simulink model "TCT_and_SUDOKU"  (R2025a)
settings: Solver=VariableStepAuto  StartTime=0.0  StopTime=1  RelTol=1e-3
libraries: spsDiodeLib x162, spsPVArrayLib x162, spsControlledVoltageSourceLib x2, spsCurrentMeasurementLib x2, simulink x2, spsVoltageMeasurementLib x2, sps_lib x1
(part 2 of 2)

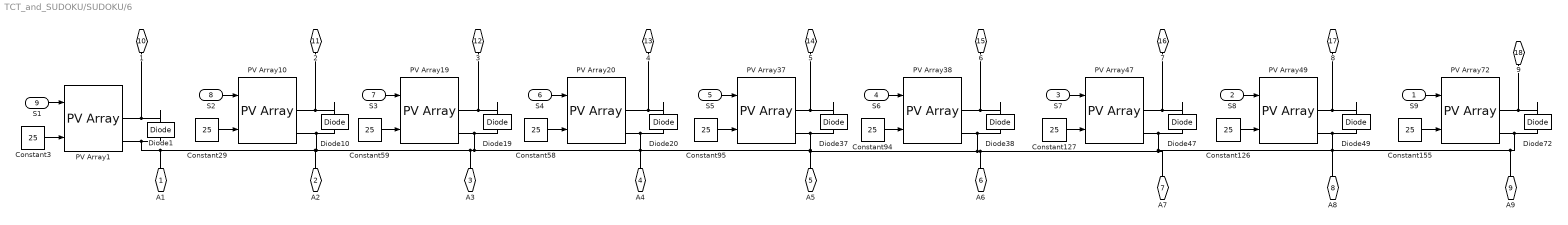
== system TCT_and_SUDOKU/SUDOKU/6 ==
  S9 : Inport
  S8 : Inport  Port=2
  S7 : Inport  Port=3
  S6 : Inport  Port=4
  S5 : Inport  Port=5
  S4 : Inport  Port=6
  S3 : Inport  Port=7
  S2 : Inport  Port=8
  S1 : Inport  Port=9
  Constant{3,29,58..59,94..95,126..127,155} (9 alike) : Constant  Value=25
  Diode{1,10,19..20,37..38,47,49,72} (9 alike) : spsDiodeLib/Diode  Ron=0.001  Lon=0  Vf=0.8  IC=0  UseSnubber=0  Rs=500  Cs=250e-9  Measurements=off
  PV Array{1,10,19..20,37..38,47,49,72} (9 alike) : spsPVArrayLib/PV Array  Npar=1  Nser=1  PlotType=array @ 1000 W/m2 & specified temperatures  S_vec="[ 1000  500  100 ]"  Temp_C_vec="[ 45 25  ]"  ModuleName=User-defined  PlotWhenSelected=off  Pm=79.2  Ncell=60  Voc=22  Isc=4.7  Vm=18  Im=4.4  beta_Voc_pc=-0.36099  alpha_Isc_pc=0.102  beta_Voc=-0.079418  alpha_Isc=0.004794  IL=4.7103  I0=1.7336e-10  nI=0.59447  Rsh=255.4401  Rs=0.29081  RobustModel=off  RobustCellTemperature=313.3991  BAL=on  Tc=1e-6  Tfilter=5e-5
  A1 : PMIOPort  Side=Left
  A2 : PMIOPort  Port=2  Side=Left
  A3 : PMIOPort  Port=3  Side=Left
  A4 : PMIOPort  Port=4  Side=Left
  A5 : PMIOPort  Port=5  Side=Left
  A6 : PMIOPort  Port=6  Side=Left
  A7 : PMIOPort  Port=7  Side=Left
  A8 : PMIOPort  Port=8  Side=Left
  A9 : PMIOPort  Port=9  Side=Left
  1 : PMIOPort  Port=10  Side=Right
  2 : PMIOPort  Port=11  Side=Right
  3 : PMIOPort  Port=12  Side=Right
  4 : PMIOPort  Port=13  Side=Right
  5 : PMIOPort  Port=14  Side=Right
  6 : PMIOPort  Port=15  Side=Right
  7 : PMIOPort  Port=16  Side=Right
  8 : PMIOPort  Port=17  Side=Right
  9 : PMIOPort  Port=18  Side=Right
  wires:
  S2/1 -> PV Array10/1
  S3/1 -> PV Array19/1
  Constant3/1 -> PV Array1/2
  S9/1 -> PV Array72/1
  Constant59/1 -> PV Array19/2
  Constant58/1 -> PV Array20/2
  Constant29/1 -> PV Array10/2
  Constant155/1 -> PV Array72/2
  S4/1 -> PV Array20/1
  S8/1 -> PV Array49/1
  Constant94/1 -> PV Array38/2
  Constant127/1 -> PV Array47/2
  S5/1 -> PV Array37/1
  Constant95/1 -> PV Array37/2
  S1/1 -> PV Array1/1
  S6/1 -> PV Array38/1
  Constant126/1 -> PV Array49/2
  S7/1 -> PV Array47/1
  connections:
  Diode10/RConn1 -- 2/RConn1 -- PV Array10/RConn1
  Diode20/RConn1 -- 4/RConn1 -- PV Array20/RConn1
  Diode19/RConn1 -- 3/RConn1 -- PV Array19/RConn1
  A6/RConn1 -- Diode47/LConn1 -- PV Array47/RConn2 -- A8/RConn1 -- Diode72/LConn1 -- PV Array72/RConn2 -- A9/RConn1 -- Diode49/LConn1 -- PV Array49/RConn2 -- A7/RConn1 -- Diode37/LConn1 -- PV Array37/RConn2 -- PV Array1/RConn2 -- Diode1/LConn1 -- A1/RConn1 -- A2/RConn1 -- PV Array10/RConn2 -- Diode10/LConn1 -- A3/RConn1 -- Diode19/LConn1 -- PV Array19/RConn2 -- A4/RConn1 -- Diode20/LConn1 -- PV Array20/RConn2 -- A5/RConn1 -- Diode38/LConn1 -- PV Array38/RConn2
  Diode47/RConn1 -- 7/RConn1 -- PV Array47/RConn1
  Diode49/RConn1 -- PV Array49/RConn1 -- 8/RConn1
  Diode1/RConn1 -- 1/RConn1 -- PV Array1/RConn1
  Diode72/RConn1 -- 9/RConn1 -- PV Array72/RConn1
  Diode37/RConn1 -- PV Array37/RConn1 -- 5/RConn1
  Diode38/RConn1 -- 6/RConn1 -- PV Array38/RConn1

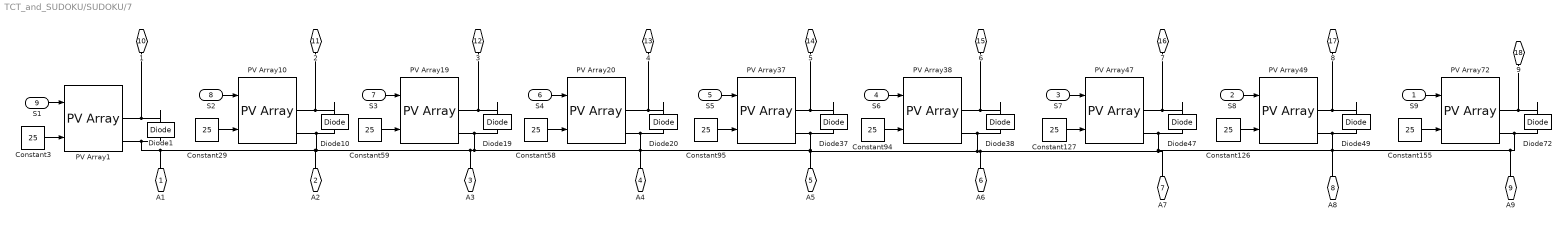
== system TCT_and_SUDOKU/SUDOKU/7 ==
  S9 : Inport
  S8 : Inport  Port=2
  S7 : Inport  Port=3
  S6 : Inport  Port=4
  S5 : Inport  Port=5
  S4 : Inport  Port=6
  S3 : Inport  Port=7
  S2 : Inport  Port=8
  S1 : Inport  Port=9
  Constant{3,29,58..59,94..95,126..127,155} (9 alike) : Constant  Value=25
  Diode{1,10,19..20,37..38,47,49,72} (9 alike) : spsDiodeLib/Diode  Ron=0.001  Lon=0  Vf=0.8  IC=0  UseSnubber=0  Rs=500  Cs=250e-9  Measurements=off
  PV Array{1,10,19..20,37..38,47,49,72} (9 alike) : spsPVArrayLib/PV Array  Npar=1  Nser=1  PlotType=array @ 1000 W/m2 & specified temperatures  S_vec="[ 1000  500  100 ]"  Temp_C_vec="[ 45 25  ]"  ModuleName=User-defined  PlotWhenSelected=off  Pm=79.2  Ncell=60  Voc=22  Isc=4.7  Vm=18  Im=4.4  beta_Voc_pc=-0.36099  alpha_Isc_pc=0.102  beta_Voc=-0.079418  alpha_Isc=0.004794  IL=4.7103  I0=1.7336e-10  nI=0.59447  Rsh=255.4401  Rs=0.29081  RobustModel=off  RobustCellTemperature=313.3991  BAL=on  Tc=1e-6  Tfilter=5e-5
  A1 : PMIOPort  Side=Left
  A2 : PMIOPort  Port=2  Side=Left
  A3 : PMIOPort  Port=3  Side=Left
  A4 : PMIOPort  Port=4  Side=Left
  A5 : PMIOPort  Port=5  Side=Left
  A6 : PMIOPort  Port=6  Side=Left
  A7 : PMIOPort  Port=7  Side=Left
  A8 : PMIOPort  Port=8  Side=Left
  A9 : PMIOPort  Port=9  Side=Left
  1 : PMIOPort  Port=10  Side=Right
  2 : PMIOPort  Port=11  Side=Right
  3 : PMIOPort  Port=12  Side=Right
  4 : PMIOPort  Port=13  Side=Right
  5 : PMIOPort  Port=14  Side=Right
  6 : PMIOPort  Port=15  Side=Right
  7 : PMIOPort  Port=16  Side=Right
  8 : PMIOPort  Port=17  Side=Right
  9 : PMIOPort  Port=18  Side=Right
  wires:
  S7/1 -> PV Array47/1
  Constant126/1 -> PV Array49/2
  S6/1 -> PV Array38/1
  S1/1 -> PV Array1/1
  Constant95/1 -> PV Array37/2
  S5/1 -> PV Array37/1
  Constant127/1 -> PV Array47/2
  Constant94/1 -> PV Array38/2
  S8/1 -> PV Array49/1
  S4/1 -> PV Array20/1
  Constant155/1 -> PV Array72/2
  Constant29/1 -> PV Array10/2
  Constant58/1 -> PV Array20/2
  Constant59/1 -> PV Array19/2
  S9/1 -> PV Array72/1
  Constant3/1 -> PV Array1/2
  S3/1 -> PV Array19/1
  S2/1 -> PV Array10/1
  connections:
  PV Array38/RConn1 -- 6/RConn1 -- Diode38/RConn1
  5/RConn1 -- PV Array37/RConn1 -- Diode37/RConn1
  PV Array72/RConn1 -- 9/RConn1 -- Diode72/RConn1
  PV Array1/RConn1 -- 1/RConn1 -- Diode1/RConn1
  8/RConn1 -- PV Array49/RConn1 -- Diode49/RConn1
  PV Array47/RConn1 -- 7/RConn1 -- Diode47/RConn1
  PV Array38/RConn2 -- Diode38/LConn1 -- A5/RConn1 -- PV Array20/RConn2 -- Diode20/LConn1 -- A4/RConn1 -- PV Array19/RConn2 -- Diode19/LConn1 -- A3/RConn1 -- Diode10/LConn1 -- PV Array10/RConn2 -- A2/RConn1 -- A1/RConn1 -- Diode1/LConn1 -- PV Array1/RConn2 -- PV Array37/RConn2 -- Diode37/LConn1 -- A7/RConn1 -- PV Array49/RConn2 -- Diode49/LConn1 -- A9/RConn1 -- PV Array72/RConn2 -- Diode72/LConn1 -- A8/RConn1 -- PV Array47/RConn2 -- Diode47/LConn1 -- A6/RConn1
  PV Array19/RConn1 -- 3/RConn1 -- Diode19/RConn1
  PV Array20/RConn1 -- 4/RConn1 -- Diode20/RConn1
  PV Array10/RConn1 -- 2/RConn1 -- Diode10/RConn1

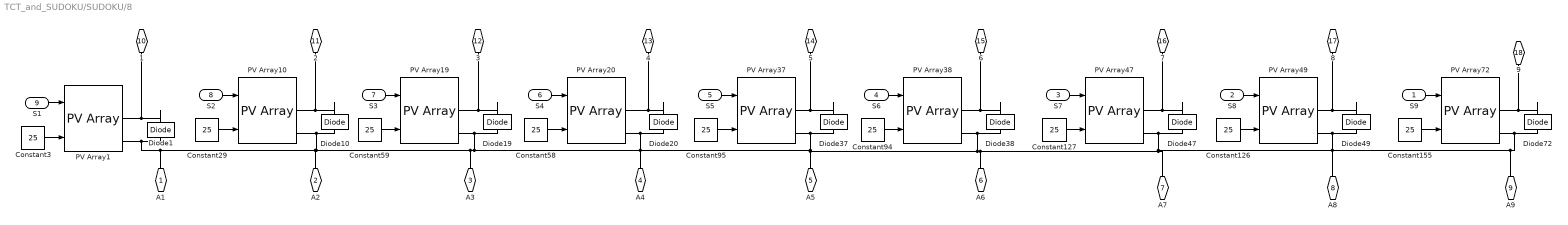
== system TCT_and_SUDOKU/SUDOKU/8 ==
  S9 : Inport
  S8 : Inport  Port=2
  S7 : Inport  Port=3
  S6 : Inport  Port=4
  S5 : Inport  Port=5
  S4 : Inport  Port=6
  S3 : Inport  Port=7
  S2 : Inport  Port=8
  S1 : Inport  Port=9
  Constant{3,29,58..59,94..95,126..127,155} (9 alike) : Constant  Value=25
  Diode{1,10,19..20,37..38,47,49,72} (9 alike) : spsDiodeLib/Diode  Ron=0.001  Lon=0  Vf=0.8  IC=0  UseSnubber=0  Rs=500  Cs=250e-9  Measurements=off
  PV Array{1,10,19..20,37..38,47,49,72} (9 alike) : spsPVArrayLib/PV Array  Npar=1  Nser=1  PlotType=array @ 1000 W/m2 & specified temperatures  S_vec="[ 1000  500  100 ]"  Temp_C_vec="[ 45 25  ]"  ModuleName=User-defined  PlotWhenSelected=off  Pm=79.2  Ncell=60  Voc=22  Isc=4.7  Vm=18  Im=4.4  beta_Voc_pc=-0.36099  alpha_Isc_pc=0.102  beta_Voc=-0.079418  alpha_Isc=0.004794  IL=4.7103  I0=1.7336e-10  nI=0.59447  Rsh=255.4401  Rs=0.29081  RobustModel=off  RobustCellTemperature=313.3991  BAL=on  Tc=1e-6  Tfilter=5e-5
  A1 : PMIOPort  Side=Left
  A2 : PMIOPort  Port=2  Side=Left
  A3 : PMIOPort  Port=3  Side=Left
  A4 : PMIOPort  Port=4  Side=Left
  A5 : PMIOPort  Port=5  Side=Left
  A6 : PMIOPort  Port=6  Side=Left
  A7 : PMIOPort  Port=7  Side=Left
  A8 : PMIOPort  Port=8  Side=Left
  A9 : PMIOPort  Port=9  Side=Left
  1 : PMIOPort  Port=10  Side=Right
  2 : PMIOPort  Port=11  Side=Right
  3 : PMIOPort  Port=12  Side=Right
  4 : PMIOPort  Port=13  Side=Right
  5 : PMIOPort  Port=14  Side=Right
  6 : PMIOPort  Port=15  Side=Right
  7 : PMIOPort  Port=16  Side=Right
  8 : PMIOPort  Port=17  Side=Right
  9 : PMIOPort  Port=18  Side=Right
  wires:
  S2/1 -> PV Array10/1
  S3/1 -> PV Array19/1
  Constant3/1 -> PV Array1/2
  S9/1 -> PV Array72/1
  Constant59/1 -> PV Array19/2
  Constant58/1 -> PV Array20/2
  Constant29/1 -> PV Array10/2
  Constant155/1 -> PV Array72/2
  S4/1 -> PV Array20/1
  S8/1 -> PV Array49/1
  Constant94/1 -> PV Array38/2
  Constant127/1 -> PV Array47/2
  S5/1 -> PV Array37/1
  Constant95/1 -> PV Array37/2
  S1/1 -> PV Array1/1
  S6/1 -> PV Array38/1
  Constant126/1 -> PV Array49/2
  S7/1 -> PV Array47/1
  connections:
  Diode10/RConn1 -- 2/RConn1 -- PV Array10/RConn1
  Diode20/RConn1 -- 4/RConn1 -- PV Array20/RConn1
  Diode19/RConn1 -- 3/RConn1 -- PV Array19/RConn1
  A6/RConn1 -- Diode47/LConn1 -- PV Array47/RConn2 -- A8/RConn1 -- Diode72/LConn1 -- PV Array72/RConn2 -- A9/RConn1 -- Diode49/LConn1 -- PV Array49/RConn2 -- A7/RConn1 -- Diode37/LConn1 -- PV Array37/RConn2 -- PV Array1/RConn2 -- Diode1/LConn1 -- A1/RConn1 -- A2/RConn1 -- PV Array10/RConn2 -- Diode10/LConn1 -- A3/RConn1 -- Diode19/LConn1 -- PV Array19/RConn2 -- A4/RConn1 -- Diode20/LConn1 -- PV Array20/RConn2 -- A5/RConn1 -- Diode38/LConn1 -- PV Array38/RConn2
  Diode47/RConn1 -- 7/RConn1 -- PV Array47/RConn1
  Diode49/RConn1 -- PV Array49/RConn1 -- 8/RConn1
  Diode1/RConn1 -- 1/RConn1 -- PV Array1/RConn1
  Diode72/RConn1 -- 9/RConn1 -- PV Array72/RConn1
  Diode37/RConn1 -- PV Array37/RConn1 -- 5/RConn1
  Diode38/RConn1 -- 6/RConn1 -- PV Array38/RConn1

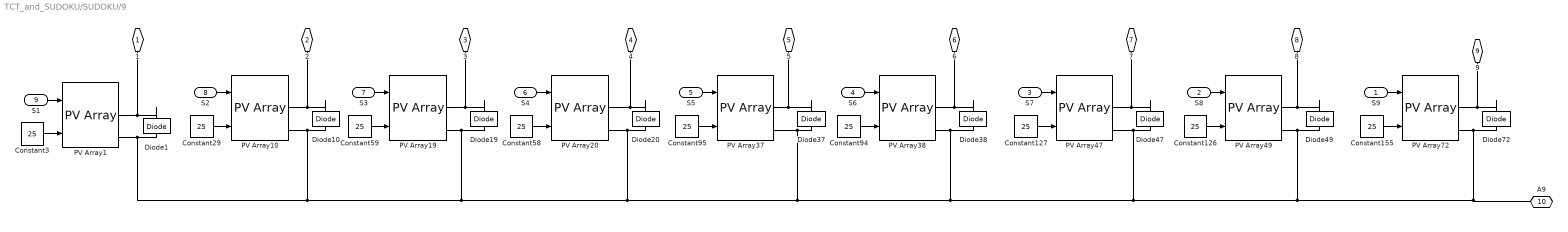
== system TCT_and_SUDOKU/SUDOKU/9 ==
  S9 : Inport
  S8 : Inport  Port=2
  S7 : Inport  Port=3
  S6 : Inport  Port=4
  S5 : Inport  Port=5
  S4 : Inport  Port=6
  S3 : Inport  Port=7
  S2 : Inport  Port=8
  S1 : Inport  Port=9
  Constant{3,29,58..59,94..95,126..127,155} (9 alike) : Constant  Value=25
  Diode{1,10,19..20,37..38,47,49,72} (9 alike) : spsDiodeLib/Diode  Ron=0.001  Lon=0  Vf=0.8  IC=0  UseSnubber=0  Rs=500  Cs=250e-9  Measurements=off
  PV Array{1,10,19..20,37..38,47,49,72} (9 alike) : spsPVArrayLib/PV Array  Npar=1  Nser=1  PlotType=array @ 1000 W/m2 & specified temperatures  S_vec="[ 1000  500  100 ]"  Temp_C_vec="[ 45 25  ]"  ModuleName=User-defined  PlotWhenSelected=off  Pm=79.2  Ncell=60  Voc=22  Isc=4.7  Vm=18  Im=4.4  beta_Voc_pc=-0.36099  alpha_Isc_pc=0.102  beta_Voc=-0.079418  alpha_Isc=0.004794  IL=4.7103  I0=1.7336e-10  nI=0.59447  Rsh=255.4401  Rs=0.29081  RobustModel=off  RobustCellTemperature=313.3991  BAL=on  Tc=1e-6  Tfilter=5e-5
  1 : PMIOPort  Side=Right
  2 : PMIOPort  Port=2  Side=Right
  3 : PMIOPort  Port=3  Side=Right
  4 : PMIOPort  Port=4  Side=Right
  5 : PMIOPort  Port=5  Side=Right
  6 : PMIOPort  Port=6  Side=Right
  7 : PMIOPort  Port=7  Side=Right
  8 : PMIOPort  Port=8  Side=Right
  9 : PMIOPort  Port=9  Side=Right
  A9 : PMIOPort  Port=10  Side=Right
  wires:
  S7/1 -> PV Array47/1
  Constant126/1 -> PV Array49/2
  S6/1 -> PV Array38/1
  S1/1 -> PV Array1/1
  Constant95/1 -> PV Array37/2
  S5/1 -> PV Array37/1
  Constant127/1 -> PV Array47/2
  Constant94/1 -> PV Array38/2
  S8/1 -> PV Array49/1
  S4/1 -> PV Array20/1
  Constant155/1 -> PV Array72/2
  Constant29/1 -> PV Array10/2
  Constant58/1 -> PV Array20/2
  Constant59/1 -> PV Array19/2
  S9/1 -> PV Array72/1
  Constant3/1 -> PV Array1/2
  S3/1 -> PV Array19/1
  S2/1 -> PV Array10/1
  connections:
  PV Array38/RConn1 -- 6/RConn1 -- Diode38/RConn1
  5/RConn1 -- PV Array37/RConn1 -- Diode37/RConn1
  PV Array72/RConn1 -- 9/RConn1 -- Diode72/RConn1
  PV Array1/RConn1 -- 1/RConn1 -- Diode1/RConn1
  8/RConn1 -- PV Array49/RConn1 -- Diode49/RConn1
  PV Array47/RConn1 -- 7/RConn1 -- Diode47/RConn1
  PV Array19/RConn2 -- Diode19/LConn1 -- Diode1/LConn1 -- PV Array1/RConn2 -- Diode10/LConn1 -- PV Array10/RConn2 -- PV Array20/RConn2 -- Diode20/LConn1 -- PV Array38/RConn2 -- Diode38/LConn1 -- PV Array49/RConn2 -- Diode49/LConn1 -- PV Array72/RConn2 -- Diode72/LConn1 -- A9/RConn1 -- PV Array47/RConn2 -- Diode47/LConn1 -- PV Array37/RConn2 -- Diode37/LConn1
  PV Array19/RConn1 -- 3/RConn1 -- Diode19/RConn1
  PV Array20/RConn1 -- 4/RConn1 -- Diode20/RConn1
  PV Array10/RConn1 -- 2/RConn1 -- Diode10/RConn1
